simulink model "test_emplanner_cs_old"  (R2021a)
settings: Solver=ode5  StartTime=0.0  StopTime=120  FixedStep=1/1000  RelTol=1e-3
PreLoadFcn:
  | mbxruntime.callbacks.PreLoadFcn(bdroot);
PostLoadFcn:
  | mbxruntime.callbacks.PostLoadFcn(bdroot);
InitFcn:
  | mbxruntime.callbacks.InitFcn(bdroot);
StartFcn:
  | mbxruntime.callbacks.StartFcn(bdroot);
StopFcn:
  | mbxruntime.callbacks.StopFcn(bdroot);
model workspace (MAT data in the model file):
  mbox_table : object (value not decoded)
  model_closed = 0
  sim_status = 0
values from neighbouring files (symbols this model uses):
  c_factor = 43.75    [emplanner_init.m]
  cf = -175016    [emplanner_init.m]
  cr = -130634    [emplanner_init.m]
  global_path_x = [-2.7494 -1.75001774493 -0.751894634419 0.244952249347 1.24051712279 2.23479835808 3.22779585569 4.21951007764 5.20994169183 6.19909144113 7.18696009523 8.17354843293 ... (3001 elements, 3001x1)]    [global_path.mat]
  global_path_y = [18.2589 18.2589 18.2589 18.2589 18.2589 18.2589 18.2589 18.2589 18.2589 18.2589 18.2589 18.2589 ... (3001 elements, 3001x1)]    [global_path.mat]
  KD_PID_distance = 0.0    (= 0)    [emplanner_init.m]
  KD_PID_speed = 0    [emplanner_init.m]
  KI_PID_distance = 0.0    (= 0)    [emplanner_init.m]
  KI_PID_speed = 0    [emplanner_init.m]
  KP_PID_distance = 0.5    [emplanner_init.m]
  KP_PID_speed = 1.8    [emplanner_init.m]
  la = 1.265    [emplanner_init.m]
  lb = 2.947-1.265    (= 1.682)    [emplanner_init.m]
  LQR_K1 = k(:,1)'    [emplanner_init.m]
  LQR_K2 = k(:,2)'    [emplanner_init.m]
  LQR_K3 = k(:,3)'    [emplanner_init.m]
  LQR_K4 = k(:,4)'    [emplanner_init.m]
  m = 2020    [emplanner_init.m]
  rack_displacement = [-39.14 , -37.2 , -35.29 , -33.43 , -31.6 , -29.81 , -28.06 , -26.34 , -24.66 ,      -23.01 , -21.38 , -19.79 , -18.23 , -16.69 , -15.18 , -13.7 , -12.23 , -10.8 , -9.38 , -7.98 ,     -6.61 , -5.25 , -3.91 , -2.59 , -1.29 , 0 , 1.27 , 2.54 , 3.78 , 5.02 , 6.24 , 7.46 , 8.66 ,      9.86 , 11.05 , 12.24 , 13.41 , 14.59 , 15.76 , 16.92 , 18.09 , 19.25 , 20.42 , 21.59 , 22.76 ,      23.93 , 25.11 , 26 ...(+26 chars)    [emplanner_init.m]
  right_wheel_ground = [-70 ,-67.2 , -64.4 , -61.6 , -58.8 , -56 , -53.2 , -50.4 , -47.6 , -44.8 , -42 ,      -39.2 , -36.4 , -33.6 , -30.8 , -28 , -25.2 , -22.4 , -19.6 , -16.8 , -14 , -11.2 , -8.4 , -5.6 ,      -2.8 , 0 , 2.8 , 5.6 , 8.4 , 11.2 , 14 , 16.8 , 19.6 , 22.4 , 25.2 , 28 , 30.8 , 33.6 , 36.4 ,      39.2 , 42 , 44.8 , 47.6 , 50.4 , 53.2 , 56 , 58.8 , 61.6 , 64.4 , 67.2 , 70 ]    [emplanner_init.m]
  vx_break_point = zeros(1,5000)    [emplanner_init.m]
undefined symbols (not defined in the file or in its folder): aubr, DiscIntNeverNeededParam, tablebr, vubr, warningInitialVelocity, x0
libraries: PreScanSimulinkLibrary x27, simulink x19, simulink_extras x6, Solver_SF x1
(part 9 of 11)

== system test_emplanner_cs_old/Audi_A8_Sedan_2/Dynamics_Simple/Chassis/Bicycle_model_[XYZ]/X_Motion/Max RPM and zero- velocity detection/SR-Memory ==
  Signal : Inport
  Set : Inport  Port=2
  Reset : Inport  Port=3
  Constant : Constant  Value=0
  Detect Rise Positive : simulink/Logic and Bit Operations/Detect Rise Positive  vinit=0  OutDataTypeStr=uint8
  Detect Rise Positive1 : simulink/Logic and Bit Operations/Detect Rise Positive  vinit=0  OutDataTypeStr=uint8
  Manual Switch : ManualSwitch
  Manual Switch1 : ManualSwitch
  Switch : Switch  Criteria=u2 ~= 0
  Switch1 : Switch  Criteria=u2 ~= 0
  Unit Delay : UnitDelay  SampleTime=-1  HasFrameUpgradeWarning=on
  Out : Outport
  wires:
  Constant/1 -> Switch1/1
  Switch/1 -> Switch1/3
  Switch1/1 -> Unit Delay/1, Out/1
  Manual Switch1/1 -> Switch1/2
  Reset/1 -> Manual Switch1/2, Detect Rise Positive1/1
  Detect Rise Positive1/1 -> Manual Switch1/1
  Signal/1 -> Switch/1
  Unit Delay/1 -> Switch/3
  Set/1 -> Detect Rise Positive/1, Manual Switch/2
  Detect Rise Positive/1 -> Manual Switch/1
  Manual Switch/1 -> Switch/2

== matlab function test_emplanner_cs_old/Audi_A8_Sedan_1/decision&planning module/referenceline provider/MATLAB Function1 ==
  data: path_x input; path_heading output; path_y input; path_kappa output
function [path_heading,path_kappa] = fcn(path_x,path_y)
%计算path的切线方向与x轴的曲率和夹角
%原理：heading=arctan(dy/dx)
%        kappa=dheading/ds;
%       ds=(dx^2+dy^2)^0.5;
%注意角度的多值性
dx=diff(path_x);
dy=diff(path_y);
%采用dx,dy中点欧拉法，再用四象限反正切计算角度
dx_pre=[dx(1);dx];
dx_after=[dx;dx(end)];
dx_final=(dx_pre+dx_after)/2;

dy_pre=[dy(1);dy];
dy_after=[dy;dy(end)];
dy_final=(dy_pre+dy_after)/2;

ds_final=sqrt(dx_final.^2+dy_final.^2);
path_heading =atan2(dy_final,dx_final);

dheading=diff(path_heading);
dheading_pre=[dheading(1);dheading];
dheading_after=[dheading;dheading(end)];
dheading_final=dheading_pre+dheading_after/2;
%防止dheading多个2pi,假设dheading较小，用sin(dheading)近似
path_kappa=sin(dheading_final)./ds_final;

== matlab function test_emplanner_cs_old/Audi_A8_Sedan_1/decision&planning module/referenceline provider/MATLAB Function2 ==
  data: host_match_point_index input; referenceline_x_init output; global_path_x input; global_path_y input; referenceline_y_init output
function [referenceline_x_init,referenceline_y_init] = fcn(host_match_point_index,global_path_x,global_path_y)
%该函数将在全局路径上提取referenceline的未平滑的初值
%输入： host_match_point_index 自车的位置在全局路径的匹配点的编号
       %global_path_x,global_path_y 全局路径数据
%输出：referenceline_x_init,referenceline_y_init 未平滑的参考线的xy坐标

%由于global path 是每1m取一个点，所以从匹配点往后取30个点，往前取150个点即可，一共181个点
%后面的点不够的话就用前面的点补，前面的点不够的话就用后面的点补，保证总数是181个

%索引初始化
start_index = -1;
%判断后面前面的点是否足够多
if host_match_point_index - 30 < 1
    %匹配点后面的点太少了，不够30个
    start_index = 1;
elseif host_match_point_index + 150 > length(global_path_x)
    %匹配点前面的点太少了，不够150个
    start_index = length(global_path_x) - 180;
    
else
    %匹配点正常情况
    start_index = host_match_point_index - 30;
end
%提取referenceline
referenceline_x_init = global_path_x(start_index:start_index + 180);
referenceline_y_init = global_path_y(start_index:start_index + 180);

== matlab function test_emplanner_cs_old/Audi_A8_Sedan_1/decision&planning module/referenceline provider/MATLAB Function3 ==
  data: path_x input; path_heading output; path_y input; path_kappa output
function [path_heading,path_kappa] = fcn(path_x,path_y)
%计算path的切线方向与x轴的曲率和夹角
%原理：heading=arctan(dy/dx)
%        kappa=dheading/ds;
%       ds=(dx^2+dy^2)^0.5;
%注意角度的多值性
dx=diff(path_x);
dy=diff(path_y);
%采用dx,dy中点欧拉法，再用四象限反正切计算角度
dx_pre=[dx(1);dx];
dx_after=[dx;dx(end)];
dx_final=(dx_pre+dx_after)/2;

dy_pre=[dy(1);dy];
dy_after=[dy;dy(end)];
dy_final=(dy_pre+dy_after)/2;

ds_final=sqrt(dx_final.^2+dy_final.^2);
path_heading =atan2(dy_final,dx_final);

dheading=diff(path_heading);
dheading_pre=[dheading(1);dheading];
dheading_after=[dheading;dheading(end)];
dheading_final=dheading_pre+dheading_after/2;
%防止dheading多个2pi,假设dheading较小，用sin(dheading)近似
path_kappa=sin(dheading_final)./ds_final;

== matlab function test_emplanner_cs_old/Audi_A8_Sedan_2/PathFollower_Preview_1/LateralController/Calculate delta steering error/eml_delta_steering_error ==
  data: v_x_vehicle input; v_x_vehicle_Min input; t_Preview_LatCtrl input; delta_steeringwheeltotal output; v_y_vehicle input; yawrate_vehicle input; CorneringStiffness_Tyres_Front input; CorneringStiffness_Tyres_Rear input; m_vehicle_total input; inertia_z_vehicle_total input; e_Lat input size=10; Pos_x_CoG_Vehicle input; wheelbase input; RefreshCounter parameter
function delta_steeringwheeltotal = eml_delta_steering_error(v_x_vehicle,v_x_vehicle_Min,t_Preview_LatCtrl,v_y_vehicle,yawrate_vehicle,CorneringStiffness_Tyres_Front,CorneringStiffness_Tyres_Rear,m_vehicle_total,inertia_z_vehicle_total,e_Lat,Pos_x_CoG_Vehicle,wheelbase,RefreshCounter)

delta_steeringwheeltotal = emlfcn_delta_steering_error(v_x_vehicle,v_x_vehicle_Min,t_Preview_LatCtrl,v_y_vehicle,yawrate_vehicle,CorneringStiffness_Tyres_Front,CorneringStiffness_Tyres_Rear,m_vehicle_total,inertia_z_vehicle_total,e_Lat,Pos_x_CoG_Vehicle,wheelbase,RefreshCounter);

% end function

== matlab function test_emplanner_cs_old/Audi_A8_Sedan_1/decision&planning module/referenceline provider/MATLAB Function4 ==
  data: referenceline_x_init input; referenceline_x output; referenceline_y_init input; w_cost_smooth input; w_cost_length input; w_cost_ref input; x_lb input; x_ub input; y_lb input; y_ub input; referenceline_y output
function [referenceline_x,referenceline_y] = ...
    fcn(referenceline_x_init,referenceline_y_init,w_cost_smooth,w_cost_length,w_cost_ref,x_lb,x_ub,y_lb,y_ub)
%用于平滑参考线
%使用二次规划
%simulink无法直接获得自带的二次规划函数，需要从外部调用
coder.extrinsic("quadprog");
n=181;
referenceline_x=zeros(n,1);
referenceline_y=zeros(n,1);
A1=zeros(2*n-4,2*n);
A2=zeros(2*n-2,2*n);
A3=eye(2*n,2*n);
f=zeros(2*n,1);
lb=zeros(2*n,1);
ub=zeros(2*n,1);
persistent is_first_run;
persistent pre_result_x;
persistent pre_result_y;
persistent pre_referenceline_x_init;
persistent pre_referenceline_y_init;

if isempty(is_first_run)
    is_first_run =0;
    for i =1:n
        f(2*i-1)=referenceline_x_init(i);
        f(2*i)=referenceline_y_init(i);
        lb(2*i-1)=f(2*i-1)+x_lb;
        ub(2*i-1)=f(2*i-1)+x_ub;
        lb(2*i)=f(2*i)+y_lb;
        ub(2*i)=f(2*i)+y_ub;
    end

    for i=1:2:2*n-5
        A1(i,i)=1;
        A1(i,i+2)=-2;
        A1(i,i+4)=1;
        A1(i+1,i+1)=1;
        A1(i+1,i+3)=-2;
        A1(i+1,i+5)=1;
    end

    for i=1:2:2*n-3
        A2(i,i)=1;
        A2(i,i+2)=-1;
        A2(i+1,i+1)=1;
        A2(i+1,i+3)=-1;
    end

    H1=w_cost_smooth*(A1'*A1)+w_cost_length*(A2'*A2)+w_cost_ref*A3;
    H=2*H1;
    %用未平滑的参考线起点作为二次规划的迭代起点
    X0=f;
    f=-2*w_cost_ref*f;
    %二次规划求解
    X=quadprog(H,f,[],[],[],[],lb,ub,X0);
    %将结果存到referenceline中
    for i=1:n
        referenceline_x(i)=X(2*i-1);
        referenceline_y(i)=X(2*i);
    end
    pre_result_x=referenceline_x;
    pre_result_y=referenceline_y;
    pre_referenceline_x_init=referenceline_x_init;
    pre_referenceline_y_init=referenceline_y_init;
else
    if pre_referenceline_x_init(1)==referenceline_x_init(1)&&...
            pre_referenceline_y_init(1)==referenceline_y_init(1)
        %起点相同，可以认为本周期和上周期的referenceline_init一模一样，就直接复用上个周期的结果
        referenceline_x=pre_result_x;
        referenceline_y=pre_result_y;
    else
          for i =1:n
        f(2*i-1)=referenceline_x_init(i);
        f(2*i)=referenceline_y_init(i);
        lb(2*i-1)=f(2*i-1)+x_lb;
        ub(2*i-1)=f(2*i-1)+x_ub;
        lb(2*i)=f(2*i)+y_lb;
        ub(2*i)=f(2*i)+y_ub;
    end

    for i=1:2:2*n-5
        A1(i,i)=1;
        A1(i,i+2)=-2;
        A1(i,i+4)=1;
        A1(i+1,i+1)=1;
        A1(i+1,i+3)=-2;
        A1(i+1,i+5)=1;
    end

    for i=1:2:2*n-3
        A2(i,i)=1;
        A2(i,i+2)=-1;
        A2(i+1,i+1)=1;
        A2(i+1,i+3)=-1;
    end

    H1=w_cost_smooth*(A1'*A1)+w_cost_length*(A2'*A2)+w_cost_ref*A3;
    H=2*H1;
    %用未平滑的参考线起点作为二次规划的迭代起点
    X0=f;
    f=-2*w_cost_ref*f;
    %二次规划求解
    X=quadprog(H,f,[],[],[],[],lb,ub,X0);
    %将结果存到referenceline中
    for i=1:n
        referenceline_x(i)=X(2*i-1);
        referenceline_y(i)=X(2*i);
    end
    pre_result_x=referenceline_x;
    pre_result_y=referenceline_y;
    pre_referenceline_x_init=referenceline_x_init;
    pre_referenceline_y_init=referenceline_y_init;  
    end
end

== matlab function test_emplanner_cs_old/Audi_A8_Sedan_1/decision&planning module/EM Planner/calc plan start info and stitch_trajectory ==
  data: pre_trajectory_x input; plan_start_x output; pre_trajectory_y input; pre_trajectory_heading input; pre_trajectory_kappa input; pre_trajectory_velocity input; pre_trajectory_accel input; pre_trajectory_time input; current_time input; host_x input; host_y input; host_heading_xy input; host_vx input; host_vy input; host_ax input; host_ay input; plan_start_y output; plan_start_heading output; plan_start_kappa output; plan_start_vx output; plan_start_vy output; plan_start_ax output; plan_start_ay output; plan_start_time output; stitch_x output; stitch_y output; stitch_heading output; stitch_kappa output; stitch_speed output; stitch_accel output; stitch_time output
function [plan_start_x,plan_start_y,plan_start_heading,plan_start_kappa,plan_start_vx,plan_start_vy,plan_start_ax,...
    plan_start_ay,plan_start_time,stitch_x,stitch_y,stitch_heading,stitch_kappa,stitch_speed,stitch_accel,stitch_time]...
    = fcn(pre_trajectory_x,pre_trajectory_y,pre_trajectory_heading,pre_trajectory_kappa,pre_trajectory_velocity,...
    pre_trajectory_accel,pre_trajectory_time,current_time,host_x,host_y,host_heading_xy,host_vx,host_vy,host_ax,host_ay)
%该函数将计算规划起点及拼接轨迹信息
%输入：上一时刻规划结果信息，本周期绝对时间及定位信息（x,y,heading,kappa为gcs坐标，vx,vy,ax,ay为vcs坐标系）
%输出：规划起点信息（vx,vy,ax,ay为gcs坐标系）及待拼接轨迹信息（一般在上一周期轨迹的current_time+100ms,往前取20个点）
%当规划完成后，本周期的规划结果和stitch_trajectory一起拼好发给控制

%输出初始化
stitch_x=zeros(20,1);
stitch_y=zeros(20,1);
stitch_heading=zeros(20,1);
stitch_kappa=zeros(20,1);
stitch_speed=zeros(20,1);
stitch_accel=zeros(20,1);
%时间为负代表没有对应的拼接轨迹
stitch_time=ones(20,1)*-1;

%申明全局变量
persistent is_first_run;
if isempty(is_first_run)
    %代表首次运行
    is_first_run=0;
    %首次运行车辆速度为0
    plan_start_x=host_x;
    plan_start_y=host_y;
    plan_start_heading=host_heading_xy;
    plan_start_kappa=0;
    plan_start_vx=0;
    plan_start_vy=0;
    plan_start_ax=0;
    plan_start_ay=0;
    %规划起点时间为当前时间+100ms
    plan_start_time=current_time+0.1;
else
    %不是首次运行
    x_cur=host_x;
    y_cur=host_y;
    heading_cur=host_heading_xy;
    kappa_cur=0;
    %vx,xy,ax,ay要转换为gcs坐标
    vx_cur=host_vx*cos(heading_cur)-host_vy*sin(heading_cur);
    vy_cur=host_vx*sin(heading_cur)+host_vy*cos(heading_cur);
    ax_cur=host_ax*cos(heading_cur)-host_ay*sin(heading_cur);
    ay_cur=host_ax*sin(heading_cur)+host_ay*cos(heading_cur);
    %规划周期100ms
    dt=0.1;
    %非首次运行，有上一周期的轨迹，找到上一周期轨迹规划的本周期车辆应该在的位置
    for i=1:length(pre_trajectory_time)-1
        if(pre_trajectory_time(i)<=current_time)&&(pre_trajectory_time(i+1)>current_time)
            break;
        end
    end
        pre_x_desire=pre_trajectory_x(i);
        pre_y_desire=pre_trajectory_y(i);
        pre_heading_desire=pre_trajectory_heading(i);
        %计算横纵向误差
        tor=[cos(pre_heading_desire);sin(pre_heading_desire)];
        nor=[-sin(pre_heading_desire);cos(pre_heading_desire)];
        %误差向量
        d_err=[host_x;host_y]-[pre_x_desire;pre_y_desire];
        %纵向误差
        lon_err=abs(d_err'*tor);
        %横向误差
        lat_err=abs(d_err'*nor);
        %纵向大于2.5，横向大于0.5，认为控制没跟上
        if(lon_err>2.5)||(lat_err>0.5)
            %处理控制未跟上,此时采用的假设为匀加速的质点模型外推规划起点
            plan_start_x=x_cur+vx_cur*dt+0.5*ax_cur*dt*dt;
            plan_start_y=y_cur+vy_cur*dt+0.5*ay_cur*dt*dt;
            plan_start_vx=vx_cur+ax_cur*dt;
            plan_start_vy=vy_cur+ay_cur*dt;
            plan_start_heading=atan2(plan_start_vy,plan_start_vx);
            plan_start_ax=ax_cur;
            plan_start_ay=ay_cur;
            plan_start_kappa=kappa_cur;
            plan_start_time=current_time+0.1;
            return;
        else
            %表示控制能跟得上规划，开始拼接
            for j=1:length(pre_trajectory_time)-1
                if(pre_trajectory_time(j)<=(current_time+0.1))&&(pre_trajectory_time(j+1)>(current_time+0.1))
                    break;
                end
            end
            %此算法运行需要trajectory的点具有很高的密度
            plan_start_x=pre_trajectory_x(j);
            plan_start_y=pre_trajectory_y(j);
            plan_start_heading=pre_trajectory_heading(j);
            plan_start_kappa=pre_trajectory_kappa(j);
            %pre_trajectory的速度加速度是指轨迹的切向速度，加速度
            plan_start_vx=pre_trajectory_velocity(j)*cos(plan_start_heading);
            plan_start_vy=pre_trajectory_velocity(j)*sin(plan_start_heading);
            %pre_trajectory的加速度是切向加速度，想计算ax,ay还要计算法向加速度
            tor=[cos(plan_start_heading);sin(plan_start_heading)];
            nor=[-sin(plan_start_heading);cos(plan_start_heading)];
            a_tor=pre_trajectory_accel(j)*tor;
            a_nor=pre_trajectory_velocity(j)^2*plan_start_kappa*nor;
            plan_start_ax=a_tor(1)+a_nor(1);
            plan_start_ay=a_tor(2)+a_nor(2);
            plan_start_time=pre_trajectory_time(j);
            %计算拼接轨迹
            %拼接是往j开始，往前拼接20个
            %选择规划包含起点，拼接不包含起点
            %把起点去掉
            j=j-1;
            if j>20
                stitch_x=pre_trajectory_x(j-19:j);
                stitch_y=pre_trajectory_y(j-19:j);
                stitch_heading=pre_trajectory_heading(j-19:j);
                stitch_kappa=pre_trajectory_kappa(j-19:j);
                stitch_speed=pre_trajectory_velocity(j-19:j);
                stitch_accel=pre_trajectory_accel(j-19:j);
                stitch_time=pre_trajectory_time(j-19:j);
            else
                stitch_x(20-j+1:20)=pre_trajectory_x(1:j);
                stitch_y(20-j+1:20)=pre_trajectory_y(1:j);
                stitch_heading(20-j+1:20)=pre_trajectory_heading(1:j);
                stitch_kappa(20-j+1:20)=pre_trajectory_kappa(1:j);
                stitch_speed(20-j+1:20)=pre_trajectory_velocity(1:j);
                stitch_accel(20-j+1:20)=pre_trajectory_accel(1:j);
                stitch_time(20-j+1:20)=pre_trajectory_time(1:j);
            end
        end
end

== matlab function test_emplanner_cs_old/Audi_A8_Sedan_1/decision&planning module/EM Planner/MATLAB Function ==
  data: s input; l input
function  fcn(s,l)
coder.extrinsic("plot")
plot(s,l)

== matlab function test_emplanner_cs_old/Audi_A8_Sedan_1/decision&planning module/EM Planner/index2s ==
  data: path_x input; index2s output; path_y input; origin_x input; origin_y input; origin_match_point_index input
function index2s = fcn(path_x,path_y,origin_x,origin_y,origin_match_point_index)
    %该算法将计算出index与s的转换关系，index2s(i)代表当序号为i时对应的弧长s
    n=181;
    index2s=zeros(n,1);
    %下面为计算以轨迹起点为坐标原点的index2s的换算关系
    for i=2:181
        index2s(i)=sqrt((path_x(i)-path_x(i-1))^2+(path_y(i)-path_y(i-1))^2)+index2s(i-1);
    end
    %计算起点到坐标原点的弧长s0,减去s0,得到了以给点坐标原点为起点的index2s的关系
    s0=CalSFormIndex2S(index2s,path_x,path_y,origin_x,origin_y,origin_match_point_index);
    index2s=index2s-ones(n,1)*s0;
end

function s=CalSFormIndex2S(index2s,path_x,path_y,proj_x,proj_y,proj_match_point_index)
    %该函数将计算给定index2s的映射关系后，计算点（proj_x,proj_y）所对应的弧长
    %投影点与匹配点的误差向量
    vector_1=[proj_x;proj_y]-[path_x(proj_match_point_index);path_y(proj_match_point_index)];
    if proj_match_point_index<length(path_x)
        %匹配点切线处的方向向量
        vector_2=[path_x(proj_match_point_index+1);path_y(proj_match_point_index+1)]-...
            [path_x(proj_match_point_index);path_y(proj_match_point_index)];
    else
         vector_2=[path_x(proj_match_point_index);path_y(proj_match_point_index)]-...
            [path_x(proj_match_point_index-1);path_y(proj_match_point_index-1)];
    end
    if vector_1'*vector_2>0
        %投影点在匹配点前面
        s=index2s(proj_match_point_index)+sqrt(vector_1'*vector_1);
    else
        %投影点在匹配点后面
        s=index2s(proj_match_point_index)-sqrt(vector_1'*vector_1);
    end
end

== matlab function test_emplanner_cs_old/Audi_A8_Sedan_1/decision&planning module/EM Planner/obs/mine_tou1 ==
  data: x_set input; match_point_index_set output; y_set input; frenet_path_x_set input; frenet_path_y_set input; frenet_path_heading_set input; proj_x_set output; proj_y_set output; proj_heading_set output; proj_kappa_set output; frenet_path_kappa_set input
function [match_point_index_set,proj_x_set,proj_y_set,proj_heading_set,proj_kappa_set] =...
    fcn(x_set,y_set,frenet_path_x_set,frenet_path_y_set,frenet_path_heading_set,frenet_path_kappa_set)
%不知道输出集合个数，预设为128个
n=128;
match_point_index_set=ones(n,1)*nan;
proj_x_set=ones(n,1)*nan;
proj_y_set=ones(n,1)*nan;
proj_heading_set=ones(n,1)*nan;
proj_kappa_set=ones(n,1)*nan;
%申明全局变量
persistent is_first_run;
persistent pre_match_point_index_set;
persistent pre_frenet_path_x_set;
persistent pre_frenet_path_y_set;
persistent pre_frenet_path_heading_set;
persistent pre_frenet_path_kappa_set;
persistent pre_x_set;
persistent pre_y_set;
if isempty(is_first_run)
    %首次运行
    is_first_run=0;
    pre_frenet_path_x_set = frenet_path_x_set;
    pre_frenet_path_y_set = frenet_path_y_set;
    pre_frenet_path_heading_set = frenet_path_heading_set;
    pre_frenet_path_kappa_set = frenet_path_kappa_set;
    pre_match_point_index_set=ones(n,1)*nan;
    for i=1:length(x_set)
        if isnan(x_set(i))
            break;
        end
        %首次运行，从第一个点开始找
        start_search_index=1;
        %用于记录distance连续增加个数
        increase_count=0;
        min_distance=inf;%假设最小距离为无穷大
        for j=start_search_index:length(frenet_path_x_set)
            distance=(x_set(i)-frenet_path_x_set(j))^2+(y_set(i)-frenet_path_y_set(j))^2;
            if distance<min_distance
                min_distance=distance;
                match_point_index_set(i)=j;
                increase_count=0;
            else
                increase_count=increase_count+1;
            end
            if increase_count>50
                 break;
            end
        end
        %通过匹配点计算投影点
        %取出匹配点编号
        match_point_index=match_point_index_set(i);
        %取出匹配点信息
        match_point_x=frenet_path_x_set(match_point_index);
        match_point_y=frenet_path_y_set(match_point_index);
        match_point_heading=frenet_path_heading_set(match_point_index);
        match_point_kappa=frenet_path_kappa_set(match_point_index);
        %计算匹配点的位置向量和方向向量
        vector_match_point=[match_point_x;match_point_y];
        vector_match_point_direction=[cos(match_point_heading);sin(match_point_heading)];
        %待投影点的位置向量
        vector_r=[x_set(i);y_set(i)];
        %通过匹配点计算
        vector_d=vector_r-vector_match_point;
        ds=vector_d'*vector_match_point_direction;
        vector_proj_point=vector_match_point+ds*vector_match_point_direction;
        proj_heading=match_point_heading+match_point_kappa*ds;
        proj_kappa=match_point_kappa;

        %合并输出结果
        proj_x_set(i)=vector_proj_point(1);
        proj_y_set(i)=vector_proj_point(2);
        proj_heading_set(i)=proj_heading;
        proj_kappa_set(i)=proj_kappa;
     end
     %匹配点计算结果保存，供下一个计算周期使用
     pre_match_point_index_set=match_point_index_set;
     pre_x_set=x_set;
     pre_y_set=y_set;
else
    %非首次运行
    for i=1:length(x_set)
        start_search_index=pre_match_point_index_set(i);
        %判断帧与帧之间的障碍物是否为同一个
        square_dis=(x_set(i)-pre_x_set(i))^2+(y_set(i)-pre_y_set(i))^2;
        if square_dis>36
            start_search_index=nan;
        end
        %对于障碍物检测而言，当感知第一次检测到障碍物时，算法不是首次运行，此时pre_match_point_index_set的值为nan，
        %如果还用上一时刻的结果作为本周期搜索起点，会出问题，进行修改
        %声明increase_count_limit
        increase_count_limit=5;
        if isnan(start_search_index)
            %没有上个周期的结果，不能只检查5次
            increase_count_limit=50;
            %搜索起点设为1
            start_search_index=1;
        end
        %用于记录distance连续增加个数
        increase_count=0;
        %判断遍历方向
        %计算上个周期的匹配点位失，前提条件是frenet的道路信息不变，参考线模块是不变的，其他模块的参考线平滑是不断变化的，因此不能作为通用模块
        vector_pre_match_point=[frenet_path_x_set(start_search_index);frenet_path_y_set(start_search_index)];
        vector_pre_match_point_direction=...
            [cos(frenet_path_heading_set(start_search_index));sin(frenet_path_heading_set(start_search_index))];
        flag=([x_set(i);y_set(i)]-vector_pre_match_point)'*vector_pre_match_point_direction;
        min_distance=inf;%假设最小距离为无穷大
        if flag>0.001
             for j=start_search_index:length(frenet_path_x_set)
                 distance=(x_set(i)-frenet_path_x_set(j))^2+(y_set(i)-frenet_path_y_set(j))^2;
                 if distance<min_distance
                    min_distance=distance;
                    match_point_index_set(i)=j;
                    increase_count=0;
                 else
                    increase_count=increase_count+1;
                 end
                 if increase_count>increase_count_limit
                     break;
                 end
             end
        elseif flag<-0.001
            for j=start_search_index:-1:1
              distance=(x_set(i)-frenet_path_x_set(j))^2+(y_set(i)-frenet_path_y_set(j))^2;
              if distance<min_distance
                  min_distance=distance;
                  match_point_index_set(i)=j;
                  increase_count=0;
              else
                  increase_count=increase_count+1;
               end
                if increase_count>increase_count_limit
                    break;
                end
            end
        else
            match_point_index_set(i) = start_search_index;
        end
        %通过匹配点计算投影点
        %取出匹配点编号
        match_point_index=match_point_index_set(i);
        %取出匹配点信息
        match_point_x=frenet_path_x_set(match_point_index);
        match_point_y=frenet_path_y_set(match_point_index);
        match_point_heading=frenet_path_heading_set(match_point_index);
        match_point_kappa=frenet_path_kappa_set(match_point_index);
        %计算匹配点的位置向量和方向向量
        vector_match_point=[match_point_x;match_point_y];
        vector_match_point_direction=[cos(match_point_heading);sin(match_point_heading)];
        %待投影点的位置向量
        vector_r=[x_set(i);y_set(i)];
        %通过匹配点计算
        vector_d=vector_r-vector_match_point;
        ds=vector_d'*vector_match_point_direction;
        vector_proj_point=vector_match_point+ds*vector_match_point_direction;
        proj_heading=match_point_heading+match_point_kappa*ds;
        proj_kappa=match_point_kappa;
        %合并输出结果
        proj_x_set(i)=vector_proj_point(1);
        proj_y_set(i)=vector_proj_point(2);
        proj_heading_set(i)=proj_heading;
        proj_kappa_set(i)=proj_kappa;
    end
    %匹配点计算结果保存，供下一个计算周期使用
    pre_match_point_index_set=match_point_index_set;
    pre_frenet_path_x_set = frenet_path_x_set;
    pre_frenet_path_y_set = frenet_path_y_set;
    pre_frenet_path_heading_set = frenet_path_heading_set;
    pre_frenet_path_kappa_set = frenet_path_kappa_set;
    pre_x_set=x_set;
    pre_y_set=y_set;
end
end

== matlab function test_emplanner_cs_old/Audi_A8_Sedan_1/preception modulel/MATLAB Function ==
  data: host_x input; obs_x_set_gcs output; host_y input; host_heading_xy input; obs_range input; obs_theta input; obs_velocity input; obs_velocity_heading input; obs_y_set_gcs output; obs_velocity_set_gcs output; obs_heading_set_gcs output
function [obs_x_set_gcs,obs_y_set_gcs,obs_velocity_set_gcs,obs_heading_set_gcs] = fcn(host_x,host_y,host_heading_xy,obs_range,obs_theta,obs_velocity,obs_velocity_heading)
%gcs代表全局坐标系
%输入为：三个定位信息，障碍物在传感器坐标系下的极坐标：range,theta；障碍物速度大小，障碍物速度方向与x轴夹角
%输出为：障碍物在世界坐标系下的：x,y,v,v与x轴的夹角heading(夹角为障碍物的速度夹角，不是几何夹角)
%输出初始化
obs_x_set_gcs=ones(32,1)*nan;
obs_y_set_gcs=ones(32,1)*nan;
obs_velocity_set_gcs=ones(32,1)*nan;
obs_heading_set_gcs=ones(32,1)*nan;
%传感器极坐标顺时针为正，世界坐标为逆时针为正
theta_tranfer=-obs_theta*pi/180;
%传感器velocity的方向以北为0度，世界坐标以东为0度
heading_tranfer=-(obs_velocity_heading+90*ones(32,1))*pi/180;
%计算传感器与障碍物的x、y方向距离
x_tranfer=obs_range.*cos(theta_tranfer+host_heading_xy);
y_tranfer=obs_range.*sin(theta_tranfer+host_heading_xy);
%计算障碍物世界坐标
for i=1:32
    if obs_range(i)~=0
        obs_x_set_gcs(i)=x_tranfer(i)+host_x+0.4*cos(host_heading_xy);
        obs_y_set_gcs(i)=y_tranfer(i)+host_y+0.4*sin(host_heading_xy);
        obs_heading_set_gcs(i)=heading_tranfer(i);
        obs_velocity_set_gcs(i)=obs_velocity(i);
    end
end

== stateflow chart test_emplanner_cs_old/Audi_A8_Sedan_1/Chart ==
  (default) -> (junction 5)
  (junction 5) -> (junction 9)
  (junction 9) -> (junction 11) [order 1] : [i>=100]
  (junction 9) -> (junction 18) [order 2] : {
      | i=i+1;
      | }
  (junction 11) -> (junction 13) : {
      | do_planning;
      | i=1;
      | }
  (junction 13) -> (junction 15)
  (junction 18) -> (junction 20)
  (junction 20) -> (junction 22) [order 1] : [j>=10]
  (junction 20) -> (junction 27) [order 2] : {
      | j=j+1;
      | }
  (junction 22) -> (junction 25) : {
      | do_control;
      | j=1;
      | }
  (junction 25) -> (junction 27)
  (junction 27) -> (junction 30)
  data: i local =1; j local =1
  events: do_planning output FUNCTION_CALL_EVENT; do_control output FUNCTION_CALL_EVENT

== matlab function test_emplanner_cs_old/Audi_A8_Sedan_1/decision&planning module/EM Planner/cartesian2frenet/MATLAB Function1 ==
  data: x_set input; s_set output; y_set input; frenet_path_x input; frenet_path_y input; proj_x_set input; proj_y_set input; proj_heading_set input; proj_match_point_index_set input; index2s input; l_set output
function [s_set,l_set] = fcn(x_set,y_set,frenet_path_x,frenet_path_y,...
    proj_x_set,proj_y_set,proj_heading_set,proj_match_point_index_set,index2s)
%该函数计算世界坐标系下的x_set,y_set的点转换到frenet_path下的坐标s l
%输入： x_set,y_set待坐标转换的点
    %  frenet_path_x,frenet_path_y  frenet坐标轴
    %  proj_x,y,heading,kappa,index 待坐标转换点的投影点的信息
    %  inde2s  frenet_path的index与s的转换表
    n=128;
    s_set=ones(n,1)*nan;
    l_set=ones(n,1)*nan;
    for i=1:length(x_set)
        if isnan(x_set(i))
            break;
        end
        s_set(i)=CalSFormIndex2S(index2s,frenet_path_x,frenet_path_y,...
            proj_x_set(i),proj_y_set(i),proj_match_point_index_set(i));
        n_r=[-sin(proj_heading_set(i));cos(proj_heading_set(i))];
        r_h=[x_set(i);y_set(i)];
        r_r=[proj_x_set(i);proj_y_set(i)];
        l_set(i)=(r_h-r_r)'*n_r;
    end
end

function s=CalSFormIndex2S(index2s,path_x,path_y,proj_x,proj_y,proj_match_point_index)
    %该函数将计算给定index2s的映射关系后，计算点（proj_x,proj_y）所对应的弧长
    %投影点与匹配点的误差向量
    vector_1=[proj_x;proj_y]-[path_x(proj_match_point_index);path_y(proj_match_point_index)];
    if proj_match_point_index<length(path_x)
        %匹配点切线处的方向向量
        vector_2=[path_x(proj_match_point_index+1);path_y(proj_match_point_index+1)]-...
            [path_x(proj_match_point_index);path_y(proj_match_point_index)];
    else
         vector_2=[path_x(proj_match_point_index);path_y(proj_match_point_index)]-...
            [path_x(proj_match_point_index-1);path_y(proj_match_point_index-1)];
    end
    if vector_1'*vector_2>0
        %投影点在匹配点前面
        s=index2s(proj_match_point_index)+sqrt(vector_1'*vector_1);
    else
        %投影点在匹配点后面
        s=index2s(proj_match_point_index)-sqrt(vector_1'*vector_1);
    end
end

== matlab function test_emplanner_cs_old/Audi_A8_Sedan_1/decision&planning module/EM Planner/cartesian2frenet/MATLAB Function ==
  data: l_set input; s_dot_set output; vx_set input; vy_set input; proj_heading_set input; proj_kappa_set input; l_dot_set output; dl_set output
function [s_dot_set,l_dot_set,dl_set] = fcn(l_set,vx_set,vy_set,proj_heading_set,proj_kappa_set)
%该函数计算frenet坐标系的s_dot,l_dot,dl/ds
n=128;
s_dot_set=ones(n,1)*nan;
l_dot_set=ones(n,1)*nan;
dl_set=ones(n,1)*nan;
for i=1:length(l_set)
    if isnan(l_set(i))
        break;
    end
    v_h=[vx_set(i);vy_set(i)];
    n_r=[-sin(proj_heading_set(i));cos(proj_heading_set(i))];
    t_r=[cos(proj_heading_set(i));sin(proj_heading_set(i))];
    s_dot_set(i)=(v_h'*t_r)/(1-proj_kappa_set(i)*l_set(i));
    l_dot_set(i)=v_h'*n_r;
    %dl_set(i)=(1-proj_kappa_set(i)*l_set(i))*(v_h'*n_r)/(v_h'*t_r);
    %l'=l_dot/s_dot，但是如果s_dot=0不行
    if abs(s_dot_set(i))<1e-6
        dl_set(i)=0;
    else
        dl_set(i)=l_dot_set(i)/s_dot_set(i);
    end
end

== matlab function test_emplanner_cs_old/Audi_A8_Sedan_1/decision&planning module/EM Planner/cartesian2frenet/MATLAB Function2 ==
  data: ax_set input; s_dot2_set output; ay_set input; proj_heading_set input; proj_kappa_set input; l_set input; s_dot_set input; dl_set input; l_dot2_set output; ddl_set output
function [s_dot2_set,l_dot2_set,ddl_set] = fcn(ax_set,ay_set,proj_heading_set,proj_kappa_set,l_set,s_dot_set,dl_set)
n=128;
s_dot2_set=ones(n,1)*nan;
l_dot2_set=ones(n,1)*nan;
ddl_set=ones(n,1)*nan;
for i=1:length(l_set)
    if isnan(l_set(i))
        break;
    end
    a_h=[ax_set(i);ay_set(i)];
    n_r=[-sin(proj_heading_set(i));cos(proj_heading_set(i))];
    t_r=[cos(proj_heading_set(i));sin(proj_heading_set(i))];
    %近似认为dkr/ds为0，简化计算
    s_dot2_set(i) = (1/(1 - proj_kappa_set(i) * l_set(i)))* (a_h' * t_r + 2 * proj_kappa_set(i) * dl_set(i) * s_dot_set(i)^2);
    l_dot2_set(i)=a_h'*n_r-proj_kappa_set(i)*(1-proj_kappa_set(i)*l_set(i))*(s_dot_set(i)^2);
    %考虑加速度为0的情况
    if s_dot_set(i)<1e-6
        ddl_set(i)=0;
    else
        ddl_set(i)=(l_dot2_set(i)-dl_set(i)*s_dot2_set(i))/(s_dot_set(i)^2);
    end
end

== matlab function test_emplanner_cs_old/Audi_A8_Sedan_1/decision&planning module/EM Planner/obs/obs filter ==
  data: host_x input; obs_x_set_final output; host_y input; host_heading_xy input; obs_x_set_gcs input; obs_y_set_gcs input; obs_velocity_set_gcs input; obs_heading_set_gcs input; obs_y_set_final output; obs_velocity_set_final output; obs_heading_set_final output
function [obs_x_set_final,obs_y_set_final,obs_velocity_set_final,obs_heading_set_final] = fcn(host_x,host_y,host_heading_xy,obs_x_set_gcs,obs_y_set_gcs,obs_velocity_set_gcs,obs_heading_set_gcs)
%该函数筛选障碍物，纵向【-10，60】横向【-10，10】的障碍物才会被考虑
%该函数只是一种单车道的临时方法，多车道时，即使障碍物距离较远也应该被考虑
%EM planner 完全体是多车道并行计算的，每个车道都生成参考线然后并行计算出多条轨迹（c++可实现），再选择最优的轨迹作为输出
%传感器最多可以识别32个障碍物
n=32;
obs_x_set_final=ones(n,1)*nan;
obs_y_set_final=ones(n,1)*nan;
obs_velocity_set_final=ones(n,1)*nan;
obs_heading_set_final=ones(n,1)*nan;
count=1;
for i=1:length(obs_x_set_gcs)
    if isnan(obs_x_set_gcs(i))
        break;
    end
    %自车的heading的方向向量与法向量
    tor=[cos(host_heading_xy);sin(host_heading_xy)];
    nor=[-sin(host_heading_xy);cos(host_heading_xy)];
    %障碍物与自车的距离向量
    vector_obs=[obs_x_set_gcs(i);obs_y_set_gcs(i)]-[host_x;host_y];
    lon_distance=vector_obs'*tor;
    lat_distance=vector_obs'*nor;
    if (lon_distance<60)&&(lon_distance>-10)&&(lat_distance<10)&&(lat_distance>-10)
        obs_x_set_final(count)=obs_x_set_gcs(i);
        obs_y_set_final(count)=obs_y_set_gcs(i);
        obs_heading_set_final(count)=obs_heading_set_gcs(i);
        obs_velocity_set_final(count)=obs_velocity_set_gcs(i);
        count=count+1;
    end
end

== matlab function test_emplanner_cs_old/Audi_A8_Sedan_1/decision&planning module/referenceline provider/mine_tou2 ==
  data: x_set input; match_point_index_set output; y_set input; frenet_path_x_set input; frenet_path_y_set input; frenet_path_heading_set input; proj_x_set output; proj_y_set output; proj_heading_set output; proj_kappa_set output; frenet_path_kappa_set input
function [match_point_index_set,proj_x_set,proj_y_set,proj_heading_set,proj_kappa_set] =...
    fcn(x_set,y_set,frenet_path_x_set,frenet_path_y_set,frenet_path_heading_set,frenet_path_kappa_set)
%不知道输出集合个数，预设为128个
n=128;
match_point_index_set=ones(n,1)*nan;
proj_x_set=ones(n,1)*nan;
proj_y_set=ones(n,1)*nan;
proj_heading_set=ones(n,1)*nan;
proj_kappa_set=ones(n,1)*nan;
%申明全局变量
persistent is_first_run;
persistent pre_match_point_index_set;
persistent pre_frenet_path_x_set;
persistent pre_frenet_path_y_set;
persistent pre_frenet_path_heading_set;
persistent pre_frenet_path_kappa_set;
persistent pre_x_set;
persistent pre_y_set;
if isempty(is_first_run)
    %首次运行
    is_first_run=0;
    pre_frenet_path_x_set = frenet_path_x_set;
    pre_frenet_path_y_set = frenet_path_y_set;
    pre_frenet_path_heading_set = frenet_path_heading_set;
    pre_frenet_path_kappa_set = frenet_path_kappa_set;
    pre_match_point_index_set=ones(n,1)*nan;
    for i=1:length(x_set)
        if isnan(x_set(i))
            break;
        end
        %首次运行，从第一个点开始找
        start_search_index=1;
        %用于记录distance连续增加个数
        increase_count=0;
        min_distance=inf;%假设最小距离为无穷大
        for j=start_search_index:length(frenet_path_x_set)
            distance=(x_set(i)-frenet_path_x_set(j))^2+(y_set(i)-frenet_path_y_set(j))^2;
            if distance<min_distance
                min_distance=distance;
                match_point_index_set(i)=j;
                increase_count=0;
            else
                increase_count=increase_count+1;
            end
            if increase_count>50
                 break;
            end
        end
        %通过匹配点计算投影点
        %取出匹配点编号
        match_point_index=match_point_index_set(i);
        %取出匹配点信息
        match_point_x=frenet_path_x_set(match_point_index);
        match_point_y=frenet_path_y_set(match_point_index);
        match_point_heading=frenet_path_heading_set(match_point_index);
        match_point_kappa=frenet_path_kappa_set(match_point_index);
        %计算匹配点的位置向量和方向向量
        vector_match_point=[match_point_x;match_point_y];
        vector_match_point_direction=[cos(match_point_heading);sin(match_point_heading)];
        %待投影点的位置向量
        vector_r=[x_set(i);y_set(i)];
        %通过匹配点计算
        vector_d=vector_r-vector_match_point;
        ds=vector_d'*vector_match_point_direction;
        vector_proj_point=vector_match_point+ds*vector_match_point_direction;
        proj_heading=match_point_heading+match_point_kappa*ds;
        proj_kappa=match_point_kappa;

        %合并输出结果
        proj_x_set(i)=vector_proj_point(1);
        proj_y_set(i)=vector_proj_point(2);
        proj_heading_set(i)=proj_heading;
        proj_kappa_set(i)=proj_kappa;
     end
     %匹配点计算结果保存，供下一个计算周期使用
     pre_match_point_index_set=match_point_index_set;
     pre_x_set=x_set;
     pre_y_set=y_set;
else
    %非首次运行
    for i=1:length(x_set)
        start_search_index=pre_match_point_index_set(i);
        %判断帧与帧之间的障碍物是否为同一个
        square_dis=(x_set(i)-pre_x_set(i))^2+(y_set(i)-pre_y_set(i))^2;
        if square_dis>36
            start_search_index=nan;
        end
        %对于障碍物检测而言，当感知第一次检测到障碍物时，算法不是首次运行，此时pre_match_point_index_set的值为nan，
        %如果还用上一时刻的结果作为本周期搜索起点，会出问题，进行修改
        %声明increase_count_limit
        increase_count_limit=5;
        if isnan(start_search_index)
            %没有上个周期的结果，不能只检查5次
            increase_count_limit=50;
            %搜索起点设为1
            start_search_index=1;
        end
        %用于记录distance连续增加个数
        increase_count=0;
        %判断遍历方向
        %计算上个周期的匹配点位失，前提条件是frenet的道路信息不变，参考线模块是不变的，其他模块的参考线平滑是不断变化的，因此不能作为通用模块
        vector_pre_match_point=[frenet_path_x_set(start_search_index);frenet_path_y_set(start_search_index)];
        vector_pre_match_point_direction=...
            [cos(frenet_path_heading_set(start_search_index));sin(frenet_path_heading_set(start_search_index))];
        flag=([x_set(i);y_set(i)]-vector_pre_match_point)'*vector_pre_match_point_direction;
        min_distance=inf;%假设最小距离为无穷大
        if flag>0.001
             for j=start_search_index:length(frenet_path_x_set)
                 distance=(x_set(i)-frenet_path_x_set(j))^2+(y_set(i)-frenet_path_y_set(j))^2;
                 if distance<min_distance
                    min_distance=distance;
                    match_point_index_set(i)=j;
                    increase_count=0;
                 else
                    increase_count=increase_count+1;
                 end
                 if increase_count>increase_count_limit
                     break;
                 end
             end
        elseif flag<-0.001
            for j=start_search_index:-1:1
              distance=(x_set(i)-frenet_path_x_set(j))^2+(y_set(i)-frenet_path_y_set(j))^2;
              if distance<min_distance
                  min_distance=distance;
                  match_point_index_set(i)=j;
                  increase_count=0;
              else
                  increase_count=increase_count+1;
               end
                if increase_count>increase_count_limit
                    break;
                end
            end
        else
            match_point_index_set(i) = start_search_index;
        end
        %通过匹配点计算投影点
        %取出匹配点编号
        match_point_index=match_point_index_set(i);
        %取出匹配点信息
        match_point_x=frenet_path_x_set(match_point_index);
        match_point_y=frenet_path_y_set(match_point_index);
        match_point_heading=frenet_path_heading_set(match_point_index);
        match_point_kappa=frenet_path_kappa_set(match_point_index);
        %计算匹配点的位置向量和方向向量
        vector_match_point=[match_point_x;match_point_y];
        vector_match_point_direction=[cos(match_point_heading);sin(match_point_heading)];
        %待投影点的位置向量
        vector_r=[x_set(i);y_set(i)];
        %通过匹配点计算
        vector_d=vector_r-vector_match_point;
        ds=vector_d'*vector_match_point_direction;
        vector_proj_point=vector_match_point+ds*vector_match_point_direction;
        proj_heading=match_point_heading+match_point_kappa*ds;
        proj_kappa=match_point_kappa;
        %合并输出结果
        proj_x_set(i)=vector_proj_point(1);
        proj_y_set(i)=vector_proj_point(2);
        proj_heading_set(i)=proj_heading;
        proj_kappa_set(i)=proj_kappa;
    end
    %匹配点计算结果保存，供下一个计算周期使用
    pre_match_point_index_set=match_point_index_set;
    pre_frenet_path_x_set = frenet_path_x_set;
    pre_frenet_path_y_set = frenet_path_y_set;
    pre_frenet_path_heading_set = frenet_path_heading_set;
    pre_frenet_path_kappa_set = frenet_path_kappa_set;
    pre_x_set=x_set;
    pre_y_set=y_set;
end
end

== matlab function test_emplanner_cs_old/Audi_A8_Sedan_1/decision&planning module/EM Planner/mine_tou ==
  data: x_set input; match_point_index_set output; y_set input; frenet_path_x_set input; frenet_path_y_set input; frenet_path_heading_set input; proj_x_set output; proj_y_set output; proj_heading_set output; proj_kappa_set output; frenet_path_kappa_set input
function [match_point_index_set,proj_x_set,proj_y_set,proj_heading_set,proj_kappa_set] =...
    fcn(x_set,y_set,frenet_path_x_set,frenet_path_y_set,frenet_path_heading_set,frenet_path_kappa_set)
%不知道输出集合个数，预设为128个
n=128;
match_point_index_set=ones(n,1)*nan;
proj_x_set=ones(n,1)*nan;
proj_y_set=ones(n,1)*nan;
proj_heading_set=ones(n,1)*nan;
proj_kappa_set=ones(n,1)*nan;
%申明全局变量
persistent is_first_run;
persistent pre_match_point_index_set;
persistent pre_frenet_path_x_set;
persistent pre_frenet_path_y_set;
persistent pre_frenet_path_heading_set;
persistent pre_frenet_path_kappa_set;
persistent pre_x_set;
persistent pre_y_set;
if isempty(is_first_run)
    %首次运行
    is_first_run=0;
    pre_frenet_path_x_set = frenet_path_x_set;
    pre_frenet_path_y_set = frenet_path_y_set;
    pre_frenet_path_heading_set = frenet_path_heading_set;
    pre_frenet_path_kappa_set = frenet_path_kappa_set;
    pre_match_point_index_set=ones(n,1)*nan;
    for i=1:length(x_set)
        if isnan(x_set(i))
            break;
        end
        %首次运行，从第一个点开始找
        start_search_index=1;
        %用于记录distance连续增加个数
        increase_count=0;
        min_distance=inf;%假设最小距离为无穷大
        for j=start_search_index:length(frenet_path_x_set)
            distance=(x_set(i)-frenet_path_x_set(j))^2+(y_set(i)-frenet_path_y_set(j))^2;
            if distance<min_distance
                min_distance=distance;
                match_point_index_set(i)=j;
                increase_count=0;
            else
                increase_count=increase_count+1;
            end
            if increase_count>50
                 break;
            end
        end
        %通过匹配点计算投影点
        %取出匹配点编号
        match_point_index=match_point_index_set(i);
        %取出匹配点信息
        match_point_x=frenet_path_x_set(match_point_index);
        match_point_y=frenet_path_y_set(match_point_index);
        match_point_heading=frenet_path_heading_set(match_point_index);
        match_point_kappa=frenet_path_kappa_set(match_point_index);
        %计算匹配点的位置向量和方向向量
        vector_match_point=[match_point_x;match_point_y];
        vector_match_point_direction=[cos(match_point_heading);sin(match_point_heading)];
        %待投影点的位置向量
        vector_r=[x_set(i);y_set(i)];
        %通过匹配点计算
        vector_d=vector_r-vector_match_point;
        ds=vector_d'*vector_match_point_direction;
        vector_proj_point=vector_match_point+ds*vector_match_point_direction;
        proj_heading=match_point_heading+match_point_kappa*ds;
        proj_kappa=match_point_kappa;

        %合并输出结果
        proj_x_set(i)=vector_proj_point(1);
        proj_y_set(i)=vector_proj_point(2);
        proj_heading_set(i)=proj_heading;
        proj_kappa_set(i)=proj_kappa;
     end
     %匹配点计算结果保存，供下一个计算周期使用
     pre_match_point_index_set=match_point_index_set;
     pre_x_set=x_set;
     pre_y_set=y_set;
else
    %非首次运行
    for i=1:length(x_set)
        start_search_index=pre_match_point_index_set(i);
        %判断帧与帧之间的障碍物是否为同一个
        square_dis=(x_set(i)-pre_x_set(i))^2+(y_set(i)-pre_y_set(i))^2;
        if square_dis>36
            start_search_index=nan;
        end
        %对于障碍物检测而言，当感知第一次检测到障碍物时，算法不是首次运行，此时pre_match_point_index_set的值为nan，
        %如果还用上一时刻的结果作为本周期搜索起点，会出问题，进行修改
        %声明increase_count_limit
        increase_count_limit=5;
        if isnan(start_search_index)
            %没有上个周期的结果，不能只检查5次
            increase_count_limit=50;
            %搜索起点设为1
            start_search_index=1;
        end
        %用于记录distance连续增加个数
        increase_count=0;
        %判断遍历方向
        %计算上个周期的匹配点位失，前提条件是frenet的道路信息不变，参考线模块是不变的，其他模块的参考线平滑是不断变化的，因此不能作为通用模块
        vector_pre_match_point=[frenet_path_x_set(start_search_index);frenet_path_y_set(start_search_index)];
        vector_pre_match_point_direction=...
            [cos(frenet_path_heading_set(start_search_index));sin(frenet_path_heading_set(start_search_index))];
        flag=([x_set(i);y_set(i)]-vector_pre_match_point)'*vector_pre_match_point_direction;
        min_distance=inf;%假设最小距离为无穷大
        if flag>0.001
             for j=start_search_index:length(frenet_path_x_set)
                 distance=(x_set(i)-frenet_path_x_set(j))^2+(y_set(i)-frenet_path_y_set(j))^2;
                 if distance<min_distance
                    min_distance=distance;
                    match_point_index_set(i)=j;
                    increase_count=0;
                 else
                    increase_count=increase_count+1;
                 end
                 if increase_count>increase_count_limit
                     break;
                 end
             end
        elseif flag<-0.001
            for j=start_search_index:-1:1
              distance=(x_set(i)-frenet_path_x_set(j))^2+(y_set(i)-frenet_path_y_set(j))^2;
              if distance<min_distance
                  min_distance=distance;
                  match_point_index_set(i)=j;
                  increase_count=0;
              else
                  increase_count=increase_count+1;
               end
                if increase_count>increase_count_limit
                    break;
                end
            end
        else
            match_point_index_set(i) = start_search_index;
        end
        %通过匹配点计算投影点
        %取出匹配点编号
        match_point_index=match_point_index_set(i);
        %取出匹配点信息
        match_point_x=frenet_path_x_set(match_point_index);
        match_point_y=frenet_path_y_set(match_point_index);
        match_point_heading=frenet_path_heading_set(match_point_index);
        match_point_kappa=frenet_path_kappa_set(match_point_index);
        %计算匹配点的位置向量和方向向量
        vector_match_point=[match_point_x;match_point_y];
        vector_match_point_direction=[cos(match_point_heading);sin(match_point_heading)];
        %待投影点的位置向量
        vector_r=[x_set(i);y_set(i)];
        %通过匹配点计算
        vector_d=vector_r-vector_match_point;
        ds=vector_d'*vector_match_point_direction;
        vector_proj_point=vector_match_point+ds*vector_match_point_direction;
        proj_heading=match_point_heading+match_point_kappa*ds;
        proj_kappa=match_point_kappa;
        %合并输出结果
        proj_x_set(i)=vector_proj_point(1);
        proj_y_set(i)=vector_proj_point(2);
        proj_heading_set(i)=proj_heading;
        proj_kappa_set(i)=proj_kappa;
    end
    %匹配点计算结果保存，供下一个计算周期使用
    pre_match_point_index_set=match_point_index_set;
    pre_frenet_path_x_set = frenet_path_x_set;
    pre_frenet_path_y_set = frenet_path_y_set;
    pre_frenet_path_heading_set = frenet_path_heading_set;
    pre_frenet_path_kappa_set = frenet_path_kappa_set;
    pre_x_set=x_set;
    pre_y_set=y_set;
end
end

== matlab function test_emplanner_cs_old/Audi_A8_Sedan_1/decision&planning module/EM Planner/obs/cartesian2frenet1/MATLAB Function ==
  data: l_set input; s_dot_set output; vx_set input; vy_set input; proj_heading_set input; proj_kappa_set input; l_dot_set output; dl_set output
function [s_dot_set,l_dot_set,dl_set] = fcn(l_set,vx_set,vy_set,proj_heading_set,proj_kappa_set)
%该函数计算frenet坐标系的s_dot,l_dot,dl/ds
n=128;
s_dot_set=ones(n,1)*nan;
l_dot_set=ones(n,1)*nan;
dl_set=ones(n,1)*nan;
for i=1:length(l_set)
    if isnan(l_set(i))
        break;
    else
        v_h=[vx_set(i);vy_set(i)];
        n_r=[-sin(proj_heading_set(i));cos(proj_heading_set(i))];
        t_r=[cos(proj_heading_set(i));sin(proj_heading_set(i))];
        s_dot_set(i)=(v_h'*t_r)/(1-proj_kappa_set(i)*l_set(i));
        l_dot_set(i)=v_h'*n_r;
        %dl_set(i)=(1-proj_kappa_set(i)*l_set(i))*(v_h'*n_r)/(v_h'*t_r);
        %l'=l_dot/s_dot，但是如果s_dot=0不行
        if abs(s_dot_set(i))<1e-6
            dl_set(i)=0;
        else
            dl_set(i)=l_dot_set(i)/s_dot_set(i);
        end
    end
end
